simulink model "MPC564xL_FOC_SIL_PIL_REF"  (Simulink 8.1)
settings: Solver=FixedStepDiscrete  StartTime=0.0  StopTime=10  FixedStep=.01  RelTol=1e-3
libraries: BAMLIB564xL x4, simulink_extras x3
settings Model: Creator=evarshavskaya  LastModifiedBy=evarshavskaya
settings DataIOCC: ExternalInput=off  InitialState=off  LimitDataPoints=off  SaveOutput=off  SignalLogging=off  SaveTime=off
settings OptimizationCC: InlineParams=on  OptimizeModelRefInitCode=on  LifeSpan=1
settings DebuggingCC: InheritedTsInSrcMsg=none  SingleTaskRateTransMsg=error  FcnCallInpInsideContextMsg=EnableAllAsWarning  UnconnectedInputMsg=error  UnconnectedOutputMsg=error  UnconnectedLineMsg=error  UnknownTsInhSupMsg=error
settings HardwareCC: ProdLargestAtomicInteger=Long  ProdLargestAtomicFloat=Double  ProdIntDivRoundTo=Zero  ProdEndianess=BigEndian  ProdHWDeviceType=Freescale->32-bit PowerPC
settings RTWCC: SystemTargetFile=rappid564xl.tlc  MakeCommand=rappid_564xl_make_rtw  TemplateMakefile=rappid_564xl_default_tmf  PostCodeGenCommand=rappid_analyzegencode(buildInfo)  Description=RAppID Toolbox MPC564xL Code Generation Target (rappid)  ProcessScript=rappid564xl_make_rtw_hook
settings CodeAppCC: IgnoreCustomStorageClasses=off  MaxIdLength=63  CustomSymbolStrType=$N$R$M  InternalIdentifier=Classic
settings STFCustomTargetCC: CodeReplacementLibrary=ANSI_C  GenerateSampleERTMain=on  CombineOutputUpdateFcns=on  SuppressErrorStatus=on  ERTCustomFileBanners=on  SupportAbsoluteTime=off  SupportContinuousTime=off  SupportNonInlinedSFcns=off  MATLABClassNameForMDSCustomization=Simulink.SoftwareTarget.ERTCustomization  GRTInterface=off  SystemTargetFile=rappid564xl.tlc
settings ERTTargetCC: CodeReplacementLibrary=ANSI_C  MultiwordLength=2048  GenerateSampleERTMain=on  ParMdlRefBuildCompliant=off  CompOptLevelCompliant=off  ConcurrentExecutionCompliant=off  SuppressErrorStatus=on  ERTFirstTimeCompliant=off  SupportAbsoluteTime=off  ModelStepFunctionPrototypeControlCompliant=off  CPPClassGenCompliant=off  InlinedParameterPlacement=NonHierarchical  ERTCustomFileTemplate=example_file_process.tlc  ConvertIfToSwitch=off  SuppressUnreachableDefaultCases=off

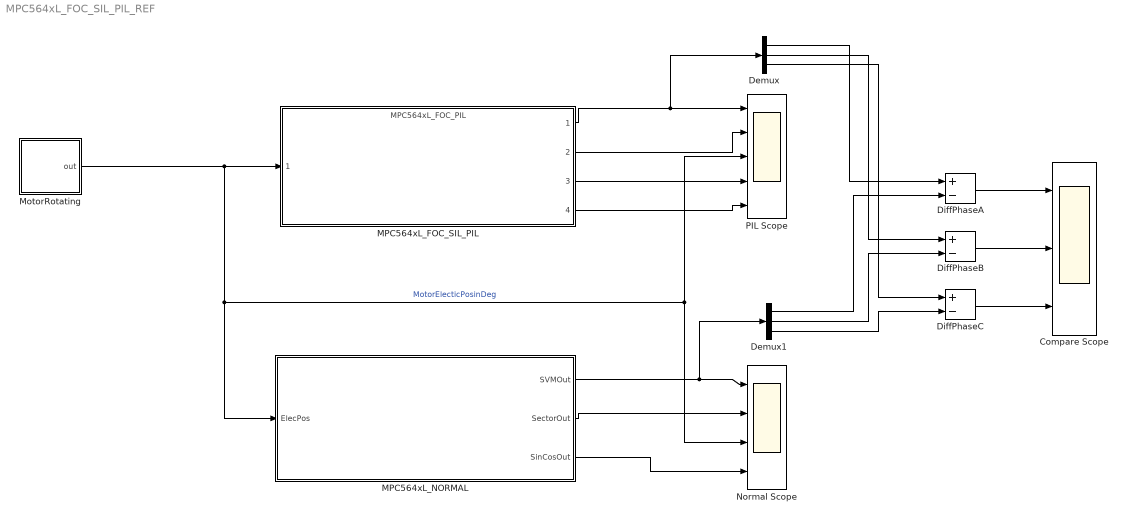
== system MPC564xL_FOC_SIL_PIL_REF ==
  Compare Scope : Scope  NumInputPorts=3
      settings: TimeRange=10  YMin=-1~-1~-1  YMax=1~1~1  SaveName=ScopeData2
  Demux : Demux  Outputs=3
  Demux1 : Demux  Outputs=3
  DiffPhaseA : Sum  Inputs=+-
  DiffPhaseB : Sum  Inputs=+-
  DiffPhaseC : Sum  Inputs=+-
  MPC564xL_FOC_SIL_PIL : ModelReference  ModelNameDialog=MPC564xL_FOC_PIL  SimulationMode=Processor-in-the-loop (PIL)  ModelReferenceVersion=1.249  CopyOfModelName=MPC564xL_FOC_PIL  DefaultDataLogging=off
  MPC564xL_NORMAL : Subsystem
  MotorRotating : Stateflow chart  TreatAsAtomicUnit=on
  Normal Scope : Scope  NumInputPorts=4
      settings: TimeRange=10  YMin=5.55112e-17~1~0~-1  YMax=1~6~350~1
  PIL Scope : Scope  NumInputPorts=5
      settings: TimeRange=10  YMin=5.55112e-017~1~0~-1~250  YMax=1~6~350~1~310  SaveName=ScopeData3
  wires:
  MPC564xL_FOC_SIL_PIL/1 -> PIL Scope/1, Demux/1
  MPC564xL_FOC_SIL_PIL/2 -> PIL Scope/2
  MPC564xL_FOC_SIL_PIL/3 -> PIL Scope/4
  MotorRotating/1(out) -> PIL Scope/3, Normal Scope/3, MPC564xL_NORMAL/1(ElecPos), MPC564xL_FOC_SIL_PIL/1  "MotorElecticPosinDeg"
  MPC564xL_FOC_SIL_PIL/4 -> PIL Scope/5
  MPC564xL_NORMAL/1(SVMOut) -> Normal Scope/1, Demux1/1
  MPC564xL_NORMAL/2(SectorOut) -> Normal Scope/2
  MPC564xL_NORMAL/3(SinCosOut) -> Normal Scope/4
  DiffPhaseA/1 -> Compare Scope/1
  Demux/1 -> DiffPhaseA/1
  Demux1/1 -> DiffPhaseA/2
  Demux/2 -> DiffPhaseB/1
  Demux1/2 -> DiffPhaseB/2
  Demux1/3 -> DiffPhaseC/2
  Demux/3 -> DiffPhaseC/1
  DiffPhaseB/1 -> Compare Scope/2
  DiffPhaseC/1 -> Compare Scope/3

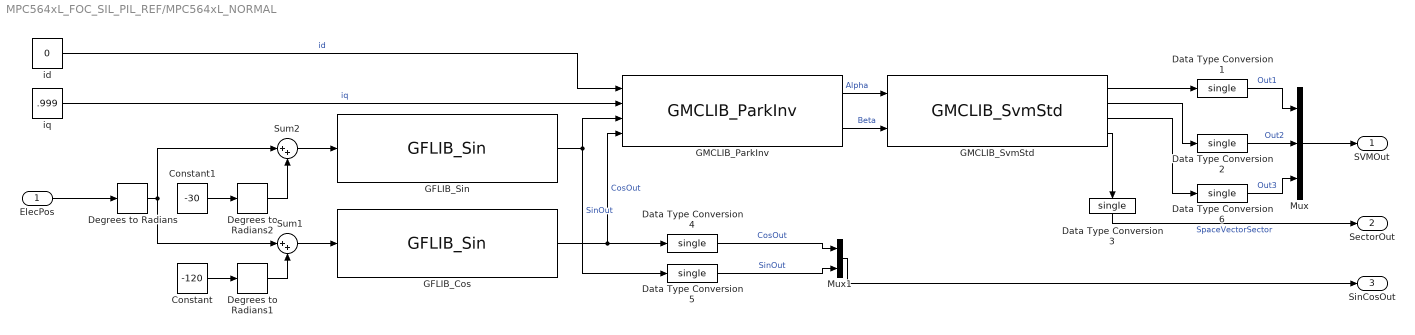
== system MPC564xL_FOC_SIL_PIL_REF/MPC564xL_NORMAL ==
  ElecPos : Inport
  Constant : Constant  Value=-120  OutDataTypeStr=single
  Constant1 : Constant  Value=-30  OutDataTypeStr=single
  Data Type Conversion{1..6} (6 alike) : DataTypeConversion  OutDataTypeStr=single
  Degrees to Radians : simulink_extras/Transformations/Degrees to Radians  SystemSampleTime=-1
  Degrees to Radians1 : simulink_extras/Transformations/Degrees to Radians  SystemSampleTime=-1
  Degrees to Radians2 : simulink_extras/Transformations/Degrees to Radians  SystemSampleTime=-1
  GFLIB_Cos : BAMLIB564xL/General Functions/GFLIB_Sin  SystemSampleTime=-1
  GFLIB_Sin : BAMLIB564xL/General Functions/GFLIB_Sin  SystemSampleTime=-1
  GMCLIB_ParkInv : BAMLIB564xL/General Motor Control Functions/GMCLIB_ParkInv  SystemSampleTime=-1
  GMCLIB_SvmStd : BAMLIB564xL/General Motor Control Functions/GMCLIB_SvmStd  SystemSampleTime=-1
  Mux : Mux  Inputs=3
  Mux1 : Mux  Inputs=2
  Sum1 : Sum  Inputs=|++
  Sum2 : Sum  Inputs=|++
  id : Constant  Value=0  OutDataTypeStr=single
  iq : Constant  Value=.999  OutDataTypeStr=single
  SVMOut : Outport
  SectorOut : Outport  Port=2
  SinCosOut : Outport  Port=3
  wires:
  GMCLIB_ParkInv/1 -> GMCLIB_SvmStd/1  "Alpha"
  GMCLIB_SvmStd/1 -> Data Type Conversion1/1
  GMCLIB_SvmStd/2 -> Data Type Conversion2/1
  GMCLIB_SvmStd/3 -> Data Type Conversion6/1
  GMCLIB_SvmStd/4 -> Data Type Conversion3/1
  id/1 -> GMCLIB_ParkInv/1  "id"
  GFLIB_Cos/1 -> GMCLIB_ParkInv/4, Data Type Conversion4/1  "CosOut"
  GFLIB_Sin/1 -> GMCLIB_ParkInv/3, Data Type Conversion5/1  "SinOut"
  iq/1 -> GMCLIB_ParkInv/2  "iq"
  Mux/1 -> SVMOut/1
  Mux1/1 -> SinCosOut/1
  Data Type Conversion1/1 -> Mux/1  "Out1"
  Data Type Conversion2/1 -> Mux/2  "Out2"
  Data Type Conversion6/1 -> Mux/3  "Out3"
  Data Type Conversion3/1 -> SectorOut/1  "SpaceVectorSector"
  Data Type Conversion5/1 -> Mux1/2  "SinOut"
  Data Type Conversion4/1 -> Mux1/1  "CosOut"
  ElecPos/1 -> Degrees to Radians/1
  Degrees to Radians/1 -> Sum2/1, Sum1/1
  Constant/1 -> Degrees to Radians1/1
  Degrees to Radians1/1 -> Sum1/2
  Constant1/1 -> Degrees to Radians2/1
  Degrees to Radians2/1 -> Sum2/2
  Sum1/1 -> GFLIB_Cos/1
  Sum2/1 -> GFLIB_Sin/1
  GMCLIB_ParkInv/2 -> GMCLIB_SvmStd/2  "Beta"

== stateflow chart MotorRotating ==
  settings: sampleTime=1/360
  state Normal
    en:out=1;
    du:out=out+1;
  Normal -> Normal : [out >= 360]
  (default) -> Normal
  data: out output single
